simulink model "msigspec_bus2"  (Simulink 6.3)
settings: Solver=FixedStepDiscrete  SolverMode=SingleTasking  StartTime=0.0  StopTime=10.0  RelTol=1e-3
undefined symbols (not defined in the file or in its folder): i
settings Model: Creator=mani  LastModifiedBy=yxiao  ExtModeAutoUpdateStatusClock=off  StrictBusMsg=ErrorLevel1
settings DataIOCC: SaveFormat=StructureWithTime  SignalLoggingName=sigsOut
settings OptimizationCC: InlineParams=on  InlineInvariantSignals=on  BufferReusableBoundary=off
settings DebuggingCC: SigSpecEnsureSampleTime=on  SolverPrmCheckMsg=none
settings HardwareCC: TargetUnknown=on

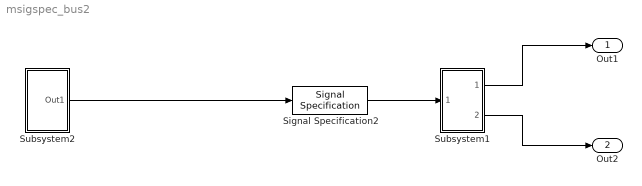
== system msigspec_bus2 ==
  Signal Specification2 : SignalSpecification
  Subsystem1 : Subsystem  TreatAsAtomicUnit=on
  Subsystem2 : Subsystem  TreatAsAtomicUnit=on
  Out1 : Outport
  Out2 : Outport  Port=2
  wires:
  Subsystem2/1(Out1) -> Signal Specification2/1
  Signal Specification2/1 -> Subsystem1/1(In1)
  Subsystem1/1(Out3) -> Out1/1
  Subsystem1/2(Out4) -> Out2/1

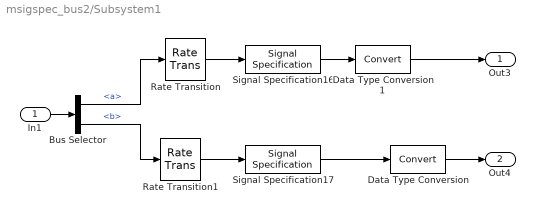
== system msigspec_bus2/Subsystem1 ==
  In1 : Inport  Port=1  LatchInput=off
  Bus Selector : BusSelector  OutputSignals=a,b
  Data Type Conversion : DataTypeConversion  OutDataTypeMode=double  SaturateOnIntegerOverflow=on  RndMeth=Zero
  Data Type Conversion1 : DataTypeConversion  OutDataTypeMode=double  SaturateOnIntegerOverflow=on  RndMeth=Zero
  Rate Transition : RateTransition  OutPortSampleTime=1
  Rate Transition1 : RateTransition  OutPortSampleTime=5
  Signal Specification16 : SignalSpecification  Dimensions=[2,2]  SampleTime=1.0  DataType=Specify via dialog  OutScaling=2^-10
      settings: SignalType=complex
  Signal Specification17 : SignalSpecification  Dimensions=[3,3]  SampleTime=5  DataType=boolean  OutScaling=2^-10
      settings: SignalType=complex
  Out3 : Outport
  Out4 : Outport  Port=2
  wires:
  Bus Selector/1 -> Rate Transition/1  "<a>"
  Bus Selector/2 -> Rate Transition1/1  "<b>"
  Data Type Conversion/1 -> Out4/1
  Data Type Conversion1/1 -> Out3/1
  Signal Specification16/1 -> Data Type Conversion1/1
  Signal Specification17/1 -> Data Type Conversion/1
  In1/1 -> Bus Selector/1
  Rate Transition/1 -> Signal Specification16/1
  Rate Transition1/1 -> Signal Specification17/1

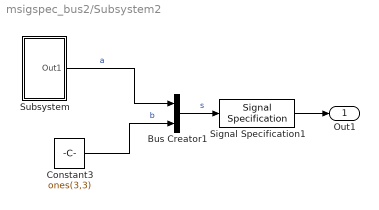
== system msigspec_bus2/Subsystem2 ==
  Bus Creator1 : BusCreator  Inputs=2
  Constant3 : Constant  Value=ones(3,3)
  Signal Specification1 : SignalSpecification
  Subsystem : Subsystem  TreatAsAtomicUnit=on
  Out1 : Outport
  wires:
  Bus Creator1/1 -> Signal Specification1/1  "s"
  Subsystem/1(Out1) -> Bus Creator1/1  "a"
  Constant3/1 -> Bus Creator1/2  "b"
  Signal Specification1/1 -> Out1/1

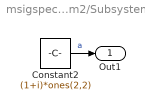
== system msigspec_bus2/Subsystem2/Subsystem ==
  Constant2 : Constant  Value=(1+i)*ones(2,2)
  Out1 : Outport
  wires:
  Constant2/1 -> Out1/1  "a"
